simulink model "GFM1MW"  (R2024b)
settings: Solver=VariableStepAuto  StartTime=0.0  StopTime=0.5  FixedStep=0.001  MaxStep=1e-3  RelTol=1e-3
values from neighbouring files (symbols this model uses):
  Cf = 6.1509e-05    [GFM1MWParameters.m]
  fbase = 50    [GFM1MWParameters.m]
  Kffi = 0.9    [GFM1MWParameters.m]
  Kffv = 0.9    [GFM1MWParameters.m]
  Kicc = Rf/Ti    (= 50)    [GFM1MWParameters.m]
  Kiq = 0.007    [GFM1MWParameters.m]
  Kivc = k*z    [GFM1MWParameters.m]
  Kpcc = (Lf1+Lf2)/Ti    (= 3.941325)    [GFM1MWParameters.m]
  Kpvc = k    [GFM1MWParameters.m]
  Lf1 = 6.8943e-04    (= 0.00068943)    [GFM1MWParameters.m]
  Lf2 = 9.8835e-05    [GFM1MWParameters.m]
  Lth = Xth/(2*pi*fbase)    [GFM1MWParameters.m]
  Mp = (2*pi*df)/(2*Pnom)    (= 3.41477462347e-06)    [GFM1MWParameters.m]
  Nq = (Vref*dV*2)/(2*Qnom)    [GFM1MWParameters.m]
  Ppowerstep = 0e6    (= 0)    [GFM1MWParameters.m]
  Pref = 0.5e6    (= 500000)    [GFM1MWParameters.m]
  Qpowerstep = 0e6    (= 0)    [GFM1MWParameters.m]
  Qref = 0.1e6    (= 100000)    [GFM1MWParameters.m]
  Rf = 0.01    [GFM1MWParameters.m]
  Rfc = 0.3450    (= 0.345)    [GFM1MWParameters.m]
  Rth = Zth/sqrt(XtoR*XtoR+1)    [GFM1MWParameters.m]
  Rvir = 0.0293    [GFM1MWParameters.m]
  Tactivepowerstep = 1.0    (= 1)    [GFM1MWParameters.m]
  Treactivepowerstep = 1.0    (= 1)    [GFM1MWParameters.m]
  Vbase = 690    [GFM1MWParameters.m]
  Vdc = 1300    [GFM1MWParameters.m]
  Vref = Vbase*sqrt(2)/sqrt(3)    [GFM1MWParameters.m]
  w = 2*pi*fbase    (= 314.159265359)    [GFM1MWParameters.m]
  Xvir = 0.0384    [GFM1MWParameters.m]
libraries: spsSeriesRLCBranchLib x15, slpidlib x4, spsGroundLib x4, dspstat3 x4, spsabctodq0Lib x4, spsThreePhaseVIMeasurementLib x3, spsFirstOrderFilterLib x2, spsThreePhaseParallelRLCLoadLib x2, spsdq0toabcLib x1, spsDCVoltageSourceLib x1, spsPLLLib x1, spsPWMGenerator2LevelLib x1
settings Model: Creator=alexs  LastModifiedBy=sproj
settings SolverCC: ZeroCrossAlgorithm=Adaptive
settings DebuggingCC: MaskedZcDiagnostic=none  IgnoredZcDiagnostic=none

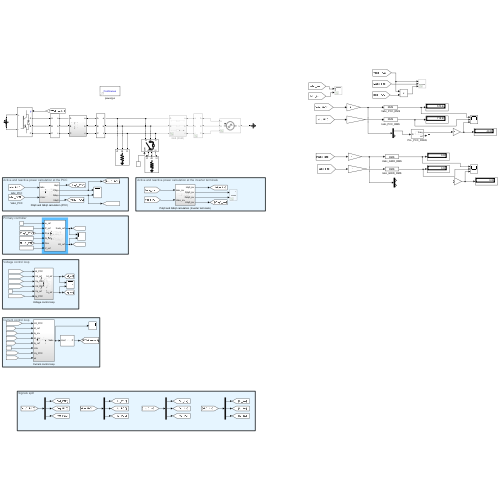
[thumbnail: Simulink's stored preview of the top-level diagram]
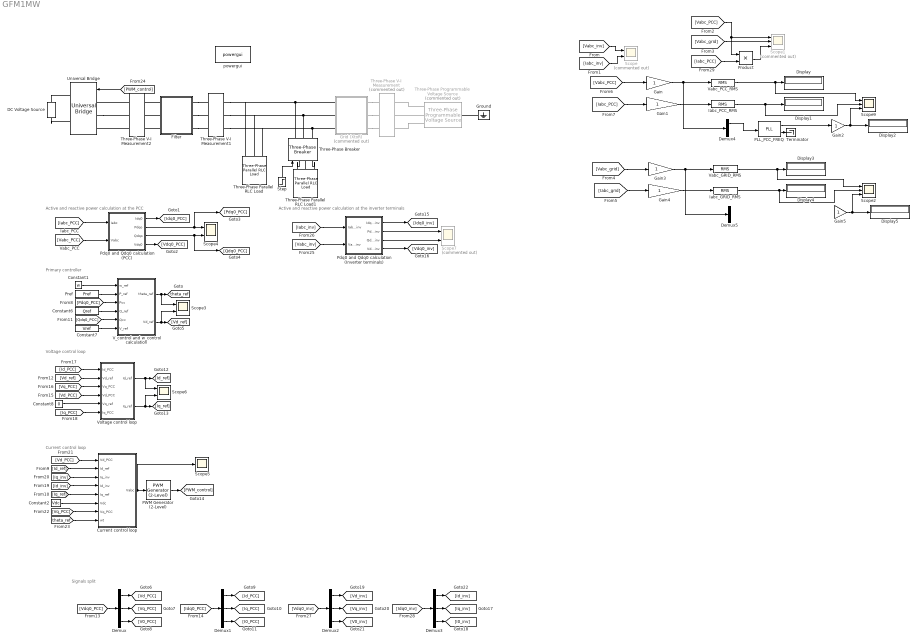
== system GFM1MW ==
  note: Active and reactive power calculation at the inverter terminals
  note: Voltage control loop
  note: Primary controller
  note: Active and reactive power calculation at the PCC
  note: Signals split
  note: Current control loop
  Constant1 : Constant  Value=w
  Constant2 : Constant  Value=Vdc
  Constant6 : Constant  Value=Qref
  Constant7 : Constant  Value=Vref
  Constant8 : Constant  Value=0
  Current control loop : Subsystem
  DC Voltage Source : spsDCVoltageSourceLib/DC Voltage Source  Amplitude=Vdc  Measurements=None
  Demux{,1..3} (4 alike) : Demux  Outputs=3
  Demux4 : Demux  Outputs=2
  Demux5 : Demux  Outputs=2
  Display{,1..5} (6 alike) : Display
      settings: Format=bank
  Filter : Subsystem
  Gain{,1..5} (6 alike) : Gain
  Grid (XtoR) : Subsystem  Commented=on
  Ground : spsGroundLib/Ground  LConnTagsString=a
  Iabc_GRID_RMS : dspstat3/RMS  run=off  directionMode=Each column  dimension=1  InputProcessing=Columns as channels (frame based)  reset_popup=None
  Iabc_PCC_RMS : dspstat3/RMS  run=off  directionMode=Each column  dimension=1  InputProcessing=Columns as channels (frame based)  reset_popup=None
  PLL_PCC_FREQ : spsPLLLib/PLL  Fmin=45  Par_Init=[0, 50]  ParK=[180, 3200, 1]  TcD=1e-4  MaxRateChangeFreq=12  FilterCutOffFreq=25  Ts=0  AGC=on
      settings: LibrarySourceBlock=sps_lib/Control/PLL
  PWM Generator (2-Level) : spsPWMGenerator2LevelLib/PWM Generator (2-Level)  ModulatorType=Three-phase bridge (6 pulses)  ModulatorMode=Unsynchronized  Fc=fsw  Pc=0  nF=27  MinMax="[ -1  1]"  SamplingTechnique=Natural  ModulatingSignals=off  m=0.8  Freq=60  Phase=0  Ts=1e-6  ShowCarrierOutport=off
  Pdq0 and Qdq0 calculation (Inverter terminals) : Subsystem
  Pdq0 and Qdq0 calculation (PCC) : Subsystem
  Pref : Constant  Value=Pref
  Product : Product
  Scope : Scope  Commented=on  NumInputPorts=2
  Scope1 : Scope  Commented=on  NumInputPorts=3
  Scope2 : Scope  NumInputPorts=3
  Scope3 : Scope  NumInputPorts=2
  Scope4 : Scope  NumInputPorts=2
  Scope5 : Scope
  Scope6 : Scope  NumInputPorts=2
  Scope7 : Scope  Commented=on  NumInputPorts=2
  Scope9 : Scope  NumInputPorts=3
  Step : Step  Time=0.1  SampleTime=0
  Terminator : Terminator
  Three-Phase Parallel RLC Load : spsThreePhaseParallelRLCLoadLib/Three-Phase Parallel RLC Load  LConnTagsString=A|B|C  Configuration=Y (grounded)  NominalVoltage=Vbase  Vabc=[1e3 1e3 1e3]  Vabcp=[1e3 1e3 1e3]  NominalFrequency=fbase  UnbalancedPower=off  ActivePower=Pref  InductivePower=Qload  CapacitivePower=0  Pabc=[10e3 9e3 11e3]  QLabc=[100 90 110]  QCabc=[100 90 110]  Pabcp=[10e3 9e3 11e3]  QLabcp=[100 90 110]  QCabcp=[100 90 110]  Measurements=None  LoadType=constant Z
  Three-Phase Parallel RLC Load1 : spsThreePhaseParallelRLCLoadLib/Three-Phase Parallel RLC Load  LConnTagsString=A|B|C  Configuration=Y (grounded)  NominalVoltage=Vbase  Vabc=[1e3 1e3 1e3]  Vabcp=[1e3 1e3 1e3]  NominalFrequency=fbase  UnbalancedPower=off  ActivePower=1e5  InductivePower=Qload  CapacitivePower=0  Pabc=[10e3 9e3 11e3]  QLabc=[100 90 110]  QCabc=[100 90 110]  Pabcp=[10e3 9e3 11e3]  QLabcp=[100 90 110]  QCabcp=[100 90 110]  Measurements=None  LoadType=constant Z
  Three-Phase Programmable Voltage Source : spsThreePhaseProgrammableVoltageSourceLib/Three-Phase Programmable Voltage Source  Commented=on  PositiveSequence="[Vbase  90 fbase]"  VariationEntity=Amplitude  VariationType=Step  VariationTypeAlt=Step  VariationStep=-0.12  VariationRate=10  VariationMagnitude=0.3  VariationFrequency=2  VariationTiming=[1 3]  VariationPhaseA=off  Amplitudes=[1 0.8 1.2 1.0]  TimeValues=[0 0.1 0.15 0.2]  HarmonicGeneration=off  HarmonicA=[3 0.2 -25 0]  HarmonicB=[2 0.15 35 2]  Timing="[0.05  3]"  BusType=swing  Pref=0  Qref=0  Qmin=-inf  Qmax=inf
  Three-Phase V-I Measurement : spsThreePhaseVIMeasurementLib/Three-Phase V-I Measurement  Commented=on  VoltageMeasurement=phase-to-ground  SetLabelV=on  LabelV=Vabc_grid  Vpu=off  VpuLL=off  CurrentMeasurement=yes  SetLabelI=on  LabelI=Iabc_grid  Ipu=off  Pbase=10000  Vbase=Vac  OutputType=Complex  PhasorSimulation=off  PSBequivalent=0
  Three-Phase V-I Measurement1 : spsThreePhaseVIMeasurementLib/Three-Phase V-I Measurement  VoltageMeasurement=phase-to-ground  SetLabelV=on  LabelV=Vabc_PCC  Vpu=off  VpuLL=off  CurrentMeasurement=yes  SetLabelI=on  LabelI=Iabc_PCC  Ipu=off  Pbase=10000  Vbase=Vac  OutputType=Complex  PhasorSimulation=off  PSBequivalent=0
  Three-Phase V-I Measurement2 : spsThreePhaseVIMeasurementLib/Three-Phase V-I Measurement  VoltageMeasurement=phase-to-ground  SetLabelV=on  LabelV=Vabc_inv  Vpu=off  VpuLL=off  CurrentMeasurement=yes  SetLabelI=on  LabelI=Iabc_inv  Ipu=off  Pbase=10000  Vbase=Vac  OutputType=Complex  PhasorSimulation=off  PSBequivalent=0
  Three-Phase Breaker : spsThreePhaseBreakerLib/Three-Phase Breaker  InitialState=open  SwitchA=on  SwitchB=on  SwitchC=on  SwitchTimes="[1/60  5/60]"  External=on  BreakerResistance=0.01  SnubberResistance=1e6  SnubberCapacitance=inf  Measurements=None
  Universal Bridge : spsUniversalBridgeLib/Universal Bridge  Arms=3  SnubberResistance=1e5  SnubberCapacitance=inf  Device=IGBT / Diodes  Ron=0  Lon=0  ForwardVoltages="[  0  0  ]"  ForwardVoltage=0  GTOparameters=[ 10e-6 , 20e-6 ]  IGBTparameters=[ 1e-6 , 2e-6 ]  Measurements=None  Measurements_2=None  converterType=Rectifier
  V_control and w_control calculation : Subsystem
  Vabc_GRID_RMS : dspstat3/RMS  run=off  directionMode=Each column  dimension=1  InputProcessing=Columns as channels (frame based)  reset_popup=None
  Vabc_PCC_RMS : dspstat3/RMS  run=off  directionMode=Each column  dimension=1  InputProcessing=Columns as channels (frame based)  reset_popup=None
  Voltage control loop : Subsystem
  powergui : sps_lib/powergui  Priority=1  SimulationMode=Continuous  SampleTime=50e-6  frequency=50  Iterations=50  frequencyindice=0  Pbase=100e6  ErrMax=1e-4  UnitsV=kV  UnitsW=MW  buscounter=0  FunctionMessages=off  echomessages=off  EnableUseOfTLC=off  CurrentSourceSwitches=off  DisableSnubberDevices=off  DisableRonSwitches=off  DisableVfSwitches=off  DisplayEquations=off  AutomaticDiscreteSolvers=off  SolverType=Tustin/Backward Euler (TBE)  Interpol=off  ExternalGateDelay=off  methode=off  Ts=10  x0status=blocks  SPID=on  SwTol=0  HookPort=off  NonlinearTolerance=1e-4  nMaxIteration=100  ContinueOnMaxIteration=off  RestoreLinks=warning  ResistiveCurrentMeasurement=off  Frange=[0:2:500]  Ylog=off  Xlog=on  ShowGrid=off  save=off  variable=ZData  structure=0  ZoomFFT=off  StartTime=0.0  cycles=1  DisplayStyle=1  fundamental=60  FreqAxis=off  MaxFrequency=1000  frequencyindicesteady=1  RmsSteady=1  display=off
  tag scope: theta_ref=global
  wires:
  [Vabc_inv] -> Scope/1
  [Iabc_inv] -> Scope/2
  [Vabc_grid] -> Scope1/2
  [Vabc_PCC] -> Product/1, Scope1/1
  Pdq0 and Qdq0 calculation (PCC)/1(Idq0) -> [Idq0_PCC]
  Pdq0 and Qdq0 calculation (PCC)/4(Vdq0) -> [Vdq0_PCC]
  Pdq0 and Qdq0 calculation (PCC)/2(Pdqo) -> Scope4/1, [Pdq0_PCC]
  Pdq0 and Qdq0 calculation (PCC)/3(Qdqo) -> [Qdq0_PCC], Scope4/2
  [Vabc_PCC] -> Gain/1
  [Iabc_PCC] -> Gain1/1
  [Iabc_PCC] -> Pdq0 and Qdq0 calculation (PCC)/1(Iabc)
  [Vabc_PCC] -> Pdq0 and Qdq0 calculation (PCC)/2(Vabc)
  Constant1/1 -> V_control and w_control calculation/1(w_ref)
  Pref/1 -> V_control and w_control calculation/2(P_ref)
  Constant6/1 -> V_control and w_control calculation/4(Q_ref)
  Constant7/1 -> V_control and w_control calculation/6(V_ref)
  V_control and w_control calculation/2(Vd_ref) -> Scope3/2, [Vd_ref]
  [Vdq0_PCC] -> Demux/1
  Demux/1 -> [Vd_PCC]
  Demux/2 -> [Vq_PCC]
  Demux/3 -> [V0_PCC]
  Demux1/1 -> [Id_PCC]
  [Idq0_PCC] -> Demux1/1
  Demux1/3 -> [I0_PCC]
  Demux1/2 -> [Iq_PCC]
  [Id_PCC] -> Voltage control loop/1(Id_PCC)
  [Vd_ref] -> Voltage control loop/2(Vd_ref)
  [Vq_PCC] -> Voltage control loop/3(Vq_PCC)
  [Vd_PCC] -> Voltage control loop/4(Vd_PCC)
  Constant8/1 -> Voltage control loop/5(Vq_ref)
  [Iq_PCC] -> Voltage control loop/6(Iq_PCC)
  Voltage control loop/1(Id_ref) -> Scope6/1, [Id_ref]
  Voltage control loop/2(Iq_ref) -> Scope6/2, [Iq_ref]
  [Vabc_inv] -> Pdq0 and Qdq0 calculation (Inverter terminals)/2(Vabc_inv)
  [Iabc_inv] -> Pdq0 and Qdq0 calculation (Inverter terminals)/1(Iabc_inv)
  Pdq0 and Qdq0 calculation (Inverter terminals)/1(Idq0_inv) -> [Idq0_inv]
  Pdq0 and Qdq0 calculation (Inverter terminals)/4(Vdq0_inv) -> [Vdq0_inv]
  Demux2/1 -> [Vd_inv]
  Demux3/2 -> [Iq_inv]
  Demux3/3 -> [I0_inv]
  [Idq0_inv] -> Demux3/1
  [Vdq0_inv] -> Demux2/1
  Demux2/3 -> [V0_inv]
  Demux3/1 -> [Id_inv]
  Demux2/2 -> [Vq_inv]
  Pdq0 and Qdq0 calculation (Inverter terminals)/2(Pdq0_inv) -> Scope7/1
  Pdq0 and Qdq0 calculation (Inverter terminals)/3(Qdq0_inv) -> Scope7/2
  [Vd_PCC] -> Current control loop/1(Vd_PCC)
  [Id_ref] -> Current control loop/2(Id_ref)
  [Iq_inv] -> Current control loop/3(Iq_inv)
  [Id_inv] -> Current control loop/4(Id_inv)
  [Iq_ref] -> Current control loop/5(Iq_ref)
  Constant2/1 -> Current control loop/6(Vdc)
  [Vq_PCC] -> Current control loop/7(Vq_PCC)
  [theta_ref] -> Current control loop/8(wt)
  Current control loop/1(Vabc) -> Scope5/1, PWM Generator (2-Level)/1
  [Qdq0_PCC] -> V_control and w_control calculation/5(Qcc)
  [Pdq0_PCC] -> V_control and w_control calculation/3(Pcc)
  V_control and w_control calculation/1(theta_ref) -> [theta_ref], Scope3/1
  PWM Generator (2-Level)/1 -> [PWM_control]
  Step/1 -> Three-Phase Breaker/1
  PLL_PCC_FREQ/2 -> Terminator/1
  Demux4/1 -> PLL_PCC_FREQ/1
  PLL_PCC_FREQ/1 -> Gain2/1
  Vabc_PCC_RMS/1 -> Scope9/1, Display/1
  Gain2/1 -> Display2/1, Scope9/3
  Product/1 -> Scope1/3
  Gain/1 -> Vabc_PCC_RMS/1, Demux4/1
  Gain1/1 -> Iabc_PCC_RMS/1
  Gain4/1 -> Iabc_GRID_RMS/1
  Gain5/1 -> Display5/1, Scope2/3
  [Iabc_grid] -> Gain4/1
  Iabc_GRID_RMS/1 -> Scope2/2, Display4/1
  [Vabc_grid] -> Gain3/1
  Vabc_GRID_RMS/1 -> Scope2/1, Display3/1
  Gain3/1 -> Vabc_GRID_RMS/1, Demux5/1
  [PWM_control] -> Universal Bridge/1
  [Iabc_PCC] -> Product/2
  Iabc_PCC_RMS/1 -> Scope9/2, Display1/1
  connections:
  Three-Phase Breaker/RConn2 -- Three-Phase V-I Measurement1/RConn2 -- Three-Phase Parallel RLC Load/LConn2 -- Grid (XtoR)/LConn2
  Three-Phase Programmable Voltage Source/RConn1 -- Three-Phase V-I Measurement/LConn1
  Three-Phase Programmable Voltage Source/RConn2 -- Three-Phase V-I Measurement/LConn2
  Three-Phase Programmable Voltage Source/RConn3 -- Three-Phase V-I Measurement/LConn3
  Three-Phase V-I Measurement2/LConn1 -- Universal Bridge/LConn1
  Three-Phase V-I Measurement2/LConn3 -- Universal Bridge/LConn3
  Universal Bridge/LConn2 -- Three-Phase V-I Measurement2/LConn2
  DC Voltage Source/RConn1 -- Universal Bridge/RConn1
  DC Voltage Source/LConn1 -- Universal Bridge/RConn2
  Three-Phase Parallel RLC Load1/LConn1 -- Three-Phase Breaker/LConn1
  Three-Phase Parallel RLC Load1/LConn2 -- Three-Phase Breaker/LConn2
  Three-Phase Parallel RLC Load1/LConn3 -- Three-Phase Breaker/LConn3
  Filter/RConn2 -- Three-Phase V-I Measurement1/LConn2
  Filter/RConn1 -- Three-Phase V-I Measurement1/LConn1
  Filter/RConn3 -- Three-Phase V-I Measurement1/LConn3
  Filter/LConn3 -- Three-Phase V-I Measurement2/RConn3
  Filter/LConn2 -- Three-Phase V-I Measurement2/RConn2
  Filter/LConn1 -- Three-Phase V-I Measurement2/RConn1
  Grid (XtoR)/RConn1 -- Three-Phase V-I Measurement/RConn1
  Grid (XtoR)/RConn2 -- Three-Phase V-I Measurement/RConn2
  Grid (XtoR)/RConn3 -- Three-Phase V-I Measurement/RConn3
  Three-Phase Breaker/RConn1 -- Three-Phase V-I Measurement1/RConn1 -- Three-Phase Parallel RLC Load/LConn1 -- Grid (XtoR)/LConn1
  Three-Phase Breaker/RConn3 -- Three-Phase Parallel RLC Load/LConn3 -- Three-Phase V-I Measurement1/RConn3 -- Grid (XtoR)/LConn3
  Ground/LConn1 -- Three-Phase Programmable Voltage Source/LConn1

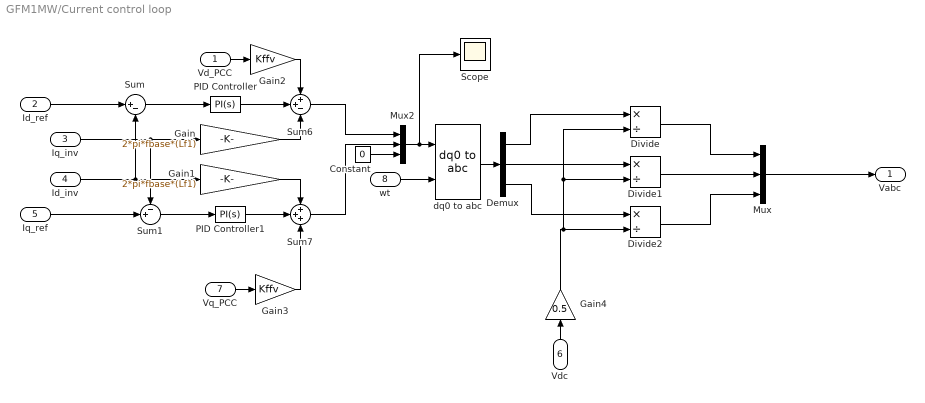
== system GFM1MW/Current control loop ==
  Vd_PCC : Inport
  Id_ref : Inport  Port=2
  Iq_inv : Inport  Port=3
  Id_inv : Inport  Port=4
  Iq_ref : Inport  Port=5
  Vdc : Inport  Port=6
  Vq_PCC : Inport  Port=7
  wt : Inport  Port=8
  Constant : Constant  Value=0
  Demux : Demux  Outputs=3
  Divide : Product  Inputs=*/
  Divide1 : Product  Inputs=*/
  Divide2 : Product  Inputs=*/
  Gain : Gain  Gain=2*pi*fbase*(Lf1)
  Gain1 : Gain  Gain=2*pi*fbase*(Lf1)
  Gain2 : Gain  Gain=Kffv
  Gain3 : Gain  Gain=Kffv
  Gain4 : Gain  Gain=0.5
  Mux : Mux  Inputs=3
  Mux2 : Mux  Inputs=3
  PID Controller : slpidlib/PID Controller  Controller=PI  Form=Parallel  TimeDomain=Continuous-time  UseExternalTs=off  SampleTime=-1  IntegratorMethod=Forward Euler  FilterMethod=Forward Euler  ControllerParametersSource=internal  P=Kpcc  I=Kicc  UseKiTs=off  D=0  UseExternalDerivativeSource=off  N=100  UseFilter=on  TunerSelectOption=Transfer Function Based (PID Tuner App)  InitialConditionSource=internal  InitialConditionForIntegrator=0  InitialConditionForFilter=0  DifferentiatorICPrevScaledInput=0  ExternalReset=none  TrackingMode=off  Kt=1  LimitOutput=off  SatLimitsSource=internal  UpperSaturationLimit=inf  LowerSaturationLimit=-inf  LinearizeAsGain=on  AntiWindupMode=none  Kb=1  LimitIntegrator=off  UpperIntegratorSaturationLimit=inf  LowerIntegratorSaturationLimit=-inf  POutMin=[]  POutMax=[]  IOutMin=[]  IOutMax=[]  DOutMin=[]  DOutMax=[]  NOutMin=[]  NOutMax=[]  SumOutMin=[]  SumOutMax=[]  SaturationOutMin=[]  SaturationOutMax=[]  PParamMin=[]  PParamMax=[]  IParamMin=[]  IParamMax=[]  DParamMin=[]  DParamMax=[]  NParamMin=[]  NParamMax=[]  KbParamMin=[]  KbParamMax=[]  KtParamMin=[]  KtParamMax=[]  KbOutMin=[]  KbOutMax=[]  KtOutMin=[]  KtOutMax=[]  IntegratorOutMin=[]  IntegratorOutMax=[]  FilterOutMin=[]  FilterOutMax=[]  SumI1OutMin=[]  SumI1OutMax=[]  SumI2OutMin=[]  SumI2OutMax=[]  SumI3OutMin=[]  SumI3OutMax=[]  SumI4OutMin=[]  SumI4OutMax=[]  SumDOutMin=[]  SumDOutMax=[]  DifferentiatorOutMin=[]  DifferentiatorOutMax=[]  FilterDiffOutCoefMin=[]  FilterDiffOutCoefMax=[]  ReciprocalOutMin=[]  ReciprocalOutMax=[]  SumDenOutMin=[]  SumDenOutMax=[]  SumNumOutMin=[]  SumNumOutMax=[]  DivideOutMin=[]  DivideOutMax=[]  UdiffTsProdOutMin=[]  UdiffTsProdOutMax=[]  NTsProdOutMin=[]  NTsProdOutMax=[]  UintegralTsProdOutMin=[]  UintegralTsProdOutMax=[]  UngainTsProdOutMin=[]  UngainTsProdOutMax=[]  ClampingZeroOutDataTypeStr=Inherit: Inherit via back propagation  ClampingZeroOutMin=[]  ClampingZeroOutMax=[]  FilterDenConstantOutDataTypeStr=Inherit: Inherit via back propagation  FilterDenConstantOutMin=[]  FilterDenConstantOutMax=[]  PCopyOutDataTypeStr=Inherit: Inherit via back propagation  PCopyOutMin=[]  PCopyOutMax=[]  NCopyOutDataTypeStr=Inherit: Inherit via back propagation  NCopyOutMin=[]  NCopyOutMax=[]  IntegratorContinuousStateAttributes=''  IntegratorStateMustResolveToSignalObject=off  IntegratorRTWStateStorageClass=Auto  FilterContinuousStateAttributes=''  FilterStateMustResolveToSignalObject=off  FilterRTWStateStorageClass=Auto  ParallelPVariant=InternalParameters  IdealPVariant=Disabled  IVariant=InternalParameters  DVariant=Disabled  IntegratorVariant=Continuous  SatVariant=Disabled  AWVariant=Passthrough  PCopyVariant=Disabled  TRVariant=Disabled  FdbkBlocksVariant=Forward  IdealPFdbkVariant=Disabled  SatFdbkVariant=Disabled  DerivativeFilterVariant=Disabled  NVariant=Disabled  NCopyVariant=Disabled_SignalSpec  FilterICVariant=Disabled  IntegratorICVariant=InternalICs  ExternalResetVariant=Disabled  TRSumVariant=Passthrough  SumFdbkVariant=Disabled  SumVariant=Sum_PI  TsampFilterVariant=InternalTs  TsampNgainVariant=Passthrough  TsampIntegralVariant=Disabled_SignalSpec  ExternalSaturationOutDataTypeStr=Inherit: Same as second input  DerivativeSourceVariant=Disabled  PreIntVariant=InternalPreInt
  PID Controller1 : slpidlib/PID Controller  Controller=PI  Form=Parallel  TimeDomain=Continuous-time  UseExternalTs=off  SampleTime=-1  IntegratorMethod=Forward Euler  FilterMethod=Forward Euler  ControllerParametersSource=internal  P=Kpcc  I=Kicc  UseKiTs=off  D=0  UseExternalDerivativeSource=off  N=100  UseFilter=on  TunerSelectOption=Transfer Function Based (PID Tuner App)  InitialConditionSource=internal  InitialConditionForIntegrator=0  InitialConditionForFilter=0  DifferentiatorICPrevScaledInput=0  ExternalReset=none  TrackingMode=off  Kt=1  LimitOutput=off  SatLimitsSource=internal  UpperSaturationLimit=inf  LowerSaturationLimit=-inf  LinearizeAsGain=on  AntiWindupMode=none  Kb=1  LimitIntegrator=off  UpperIntegratorSaturationLimit=inf  LowerIntegratorSaturationLimit=-inf  POutMin=[]  POutMax=[]  IOutMin=[]  IOutMax=[]  DOutMin=[]  DOutMax=[]  NOutMin=[]  NOutMax=[]  SumOutMin=[]  SumOutMax=[]  SaturationOutMin=[]  SaturationOutMax=[]  PParamMin=[]  PParamMax=[]  IParamMin=[]  IParamMax=[]  DParamMin=[]  DParamMax=[]  NParamMin=[]  NParamMax=[]  KbParamMin=[]  KbParamMax=[]  KtParamMin=[]  KtParamMax=[]  KbOutMin=[]  KbOutMax=[]  KtOutMin=[]  KtOutMax=[]  IntegratorOutMin=[]  IntegratorOutMax=[]  FilterOutMin=[]  FilterOutMax=[]  SumI1OutMin=[]  SumI1OutMax=[]  SumI2OutMin=[]  SumI2OutMax=[]  SumI3OutMin=[]  SumI3OutMax=[]  SumI4OutMin=[]  SumI4OutMax=[]  SumDOutMin=[]  SumDOutMax=[]  DifferentiatorOutMin=[]  DifferentiatorOutMax=[]  FilterDiffOutCoefMin=[]  FilterDiffOutCoefMax=[]  ReciprocalOutMin=[]  ReciprocalOutMax=[]  SumDenOutMin=[]  SumDenOutMax=[]  SumNumOutMin=[]  SumNumOutMax=[]  DivideOutMin=[]  DivideOutMax=[]  UdiffTsProdOutMin=[]  UdiffTsProdOutMax=[]  NTsProdOutMin=[]  NTsProdOutMax=[]  UintegralTsProdOutMin=[]  UintegralTsProdOutMax=[]  UngainTsProdOutMin=[]  UngainTsProdOutMax=[]  ClampingZeroOutDataTypeStr=Inherit: Inherit via back propagation  ClampingZeroOutMin=[]  ClampingZeroOutMax=[]  FilterDenConstantOutDataTypeStr=Inherit: Inherit via back propagation  FilterDenConstantOutMin=[]  FilterDenConstantOutMax=[]  PCopyOutDataTypeStr=Inherit: Inherit via back propagation  PCopyOutMin=[]  PCopyOutMax=[]  NCopyOutDataTypeStr=Inherit: Inherit via back propagation  NCopyOutMin=[]  NCopyOutMax=[]  IntegratorContinuousStateAttributes=''  IntegratorStateMustResolveToSignalObject=off  IntegratorRTWStateStorageClass=Auto  FilterContinuousStateAttributes=''  FilterStateMustResolveToSignalObject=off  FilterRTWStateStorageClass=Auto  ParallelPVariant=InternalParameters  IdealPVariant=Disabled  IVariant=InternalParameters  DVariant=Disabled  IntegratorVariant=Continuous  SatVariant=Disabled  AWVariant=Passthrough  PCopyVariant=Disabled  TRVariant=Disabled  FdbkBlocksVariant=Forward  IdealPFdbkVariant=Disabled  SatFdbkVariant=Disabled  DerivativeFilterVariant=Disabled  NVariant=Disabled  NCopyVariant=Disabled_SignalSpec  FilterICVariant=Disabled  IntegratorICVariant=InternalICs  ExternalResetVariant=Disabled  TRSumVariant=Passthrough  SumFdbkVariant=Disabled  SumVariant=Sum_PI  TsampFilterVariant=InternalTs  TsampNgainVariant=Passthrough  TsampIntegralVariant=Disabled_SignalSpec  ExternalSaturationOutDataTypeStr=Inherit: Same as second input  DerivativeSourceVariant=Disabled  PreIntVariant=InternalPreInt
  Scope : Scope
  Sum : Sum  Inputs=|+-
  Sum1 : Sum  Inputs=-+|
  Sum6 : Sum  Inputs=++-
  Sum7 : Sum  Inputs=+++
  dq0 to abc : spsdq0toabcLib/dq0 to abc  Alignment=Aligned with phase A axis
  Vabc : Outport
  wires:
  Gain/1 -> Sum6/3
  PID Controller1/1 -> Sum7/2
  Gain2/1 -> Sum6/1
  Iq_inv/1 -> Gain/1, Sum1/1
  Sum1/1 -> PID Controller1/1
  PID Controller/1 -> Sum6/2
  Mux2/1 -> Scope/1, dq0 to abc/1
  Id_inv/1 -> Gain1/1, Sum/2
  Vq_PCC/1 -> Gain3/1
  Sum/1 -> PID Controller/1
  Iq_ref/1 -> Sum1/2
  Gain1/1 -> Sum7/1
  Gain3/1 -> Sum7/3
  Vd_PCC/1 -> Gain2/1
  wt/1 -> dq0 to abc/2
  Id_ref/1 -> Sum/1
  Sum6/1 -> Mux2/1
  Sum7/1 -> Mux2/2
  Constant/1 -> Mux2/3
  Vdc/1 -> Gain4/1
  Mux/1 -> Vabc/1
  Gain4/1 -> Divide/2, Divide1/2, Divide2/2
  Divide2/1 -> Mux/3
  Demux/1 -> Divide/1
  Demux/2 -> Divide1/1
  Divide/1 -> Mux/1
  Demux/3 -> Divide2/1
  Divide1/1 -> Mux/2
  dq0 to abc/1 -> Demux/1

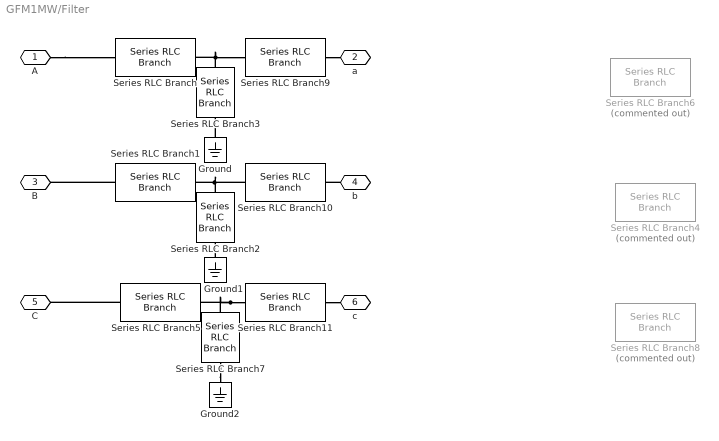
== system GFM1MW/Filter ==
  Ground : spsGroundLib/Ground  LConnTagsString=a
  Ground1 : spsGroundLib/Ground  LConnTagsString=a
  Ground2 : spsGroundLib/Ground  LConnTagsString=a
  Series RLC Branch : spsSeriesRLCBranchLib/Series RLC Branch  LConnTagsString=__new0  RConnTagsString=__new0  BranchType=RL  Resistance=Rf  Inductance=Lf1  SetiL0=off  InitialCurrent=0  Capacitance=1e-6  Setx0=off  InitialVoltage=0  Measurements=None
  Series RLC Branch1 : spsSeriesRLCBranchLib/Series RLC Branch  LConnTagsString=__new0  RConnTagsString=__new0  BranchType=RL  Resistance=Rf  Inductance=Lf1  SetiL0=off  InitialCurrent=0  Capacitance=1e-6  Setx0=off  InitialVoltage=0  Measurements=None
  Series RLC Branch10 : spsSeriesRLCBranchLib/Series RLC Branch  LConnTagsString=__new0  RConnTagsString=__new0  BranchType=L  Resistance=Rf  Inductance=Lf2  SetiL0=off  InitialCurrent=0  Capacitance=1e-6  Setx0=off  InitialVoltage=0  Measurements=None
  Series RLC Branch11 : spsSeriesRLCBranchLib/Series RLC Branch  LConnTagsString=__new0  RConnTagsString=__new0  BranchType=L  Resistance=Rf  Inductance=Lf2  SetiL0=off  InitialCurrent=0  Capacitance=1e-6  Setx0=off  InitialVoltage=0  Measurements=None
  Series RLC Branch2 : spsSeriesRLCBranchLib/Series RLC Branch  LConnTagsString=__new0  RConnTagsString=__new0  BranchType=RC  Resistance=Rfc  Inductance=1e-3  SetiL0=off  InitialCurrent=0  Capacitance=Cf  Setx0=off  InitialVoltage=0  Measurements=None
  Series RLC Branch3 : spsSeriesRLCBranchLib/Series RLC Branch  LConnTagsString=__new0  RConnTagsString=__new0  BranchType=RC  Resistance=Rfc  Inductance=1e-3  SetiL0=off  InitialCurrent=0  Capacitance=Cf  Setx0=off  InitialVoltage=0  Measurements=None
  Series RLC Branch4 : spsSeriesRLCBranchLib/Series RLC Branch  Commented=on  LConnTagsString=__new0  RConnTagsString=__new0  BranchType=L  Resistance=Rf  Inductance=Lf2  SetiL0=off  InitialCurrent=0  Capacitance=1e-6  Setx0=off  InitialVoltage=0  Measurements=None
  Series RLC Branch5 : spsSeriesRLCBranchLib/Series RLC Branch  LConnTagsString=__new0  RConnTagsString=__new0  BranchType=RL  Resistance=Rf  Inductance=Lf1  SetiL0=off  InitialCurrent=0  Capacitance=1e-6  Setx0=off  InitialVoltage=0  Measurements=None
  Series RLC Branch6 : spsSeriesRLCBranchLib/Series RLC Branch  Commented=on  LConnTagsString=__new0  RConnTagsString=__new0  BranchType=L  Resistance=Rf  Inductance=Lf2  SetiL0=off  InitialCurrent=0  Capacitance=1e-6  Setx0=off  InitialVoltage=0  Measurements=None
  Series RLC Branch7 : spsSeriesRLCBranchLib/Series RLC Branch  LConnTagsString=__new0  RConnTagsString=__new0  BranchType=RC  Resistance=Rfc  Inductance=1e-3  SetiL0=off  InitialCurrent=0  Capacitance=Cf  Setx0=off  InitialVoltage=0  Measurements=None
  Series RLC Branch8 : spsSeriesRLCBranchLib/Series RLC Branch  Commented=on  LConnTagsString=__new0  RConnTagsString=__new0  BranchType=L  Resistance=Rf  Inductance=Lf2  SetiL0=off  InitialCurrent=0  Capacitance=1e-6  Setx0=off  InitialVoltage=0  Measurements=None
  Series RLC Branch9 : spsSeriesRLCBranchLib/Series RLC Branch  LConnTagsString=__new0  RConnTagsString=__new0  BranchType=L  Resistance=Rf  Inductance=Lf2  SetiL0=off  InitialCurrent=0  Capacitance=1e-6  Setx0=off  InitialVoltage=0  Measurements=None
  A : PMIOPort  Side=Left
  a : PMIOPort  Port=2  Side=Right
  B : PMIOPort  Port=3  Side=Left
  b : PMIOPort  Port=4  Side=Right
  C : PMIOPort  Port=5  Side=Left
  c : PMIOPort  Port=6  Side=Right
  connections:
  Series RLC Branch1/LConn1 -- B/RConn1
  A/RConn1 -- Series RLC Branch/LConn1
  Ground/LConn1 -- Series RLC Branch3/RConn1
  Series RLC Branch5/LConn1 -- C/RConn1
  Series RLC Branch7/RConn1 -- Ground2/LConn1
  Ground1/LConn1 -- Series RLC Branch2/RConn1
  Series RLC Branch3/LConn1 -- Series RLC Branch9/LConn1 -- Series RLC Branch/RConn1
  b/RConn1 -- Series RLC Branch10/RConn1
  Series RLC Branch11/LConn1 -- Series RLC Branch5/RConn1 -- Series RLC Branch7/LConn1
  Series RLC Branch9/RConn1 -- a/RConn1
  Series RLC Branch10/LConn1 -- Series RLC Branch1/RConn1 -- Series RLC Branch2/LConn1
  Series RLC Branch11/RConn1 -- c/RConn1

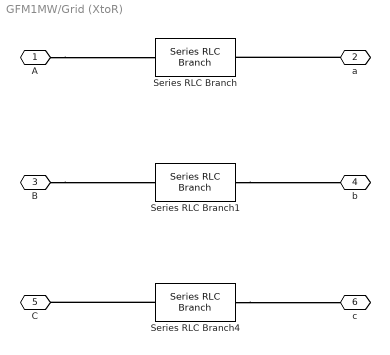
== system GFM1MW/Grid (XtoR) ==
  Series RLC Branch : spsSeriesRLCBranchLib/Series RLC Branch  LConnTagsString=__new0  RConnTagsString=__new0  BranchType=RL  Resistance=Rth  Inductance=Lth  SetiL0=off  InitialCurrent=0  Capacitance=1e-6  Setx0=off  InitialVoltage=0  Measurements=None
  Series RLC Branch1 : spsSeriesRLCBranchLib/Series RLC Branch  LConnTagsString=__new0  RConnTagsString=__new0  BranchType=RL  Resistance=Rth  Inductance=Lth  SetiL0=off  InitialCurrent=0  Capacitance=1e-6  Setx0=off  InitialVoltage=0  Measurements=None
  Series RLC Branch4 : spsSeriesRLCBranchLib/Series RLC Branch  LConnTagsString=__new0  RConnTagsString=__new0  BranchType=RL  Resistance=Rth  Inductance=Lth  SetiL0=off  InitialCurrent=0  Capacitance=1e-6  Setx0=off  InitialVoltage=0  Measurements=None
  A : PMIOPort  Side=Left
  a : PMIOPort  Port=2  Side=Right
  B : PMIOPort  Port=3  Side=Left
  b : PMIOPort  Port=4  Side=Right
  C : PMIOPort  Port=5  Side=Left
  c : PMIOPort  Port=6  Side=Right
  connections:
  B/RConn1 -- Series RLC Branch1/LConn1
  Series RLC Branch1/RConn1 -- b/RConn1
  A/RConn1 -- Series RLC Branch/LConn1
  a/RConn1 -- Series RLC Branch/RConn1
  Series RLC Branch4/RConn1 -- c/RConn1
  Series RLC Branch4/LConn1 -- C/RConn1

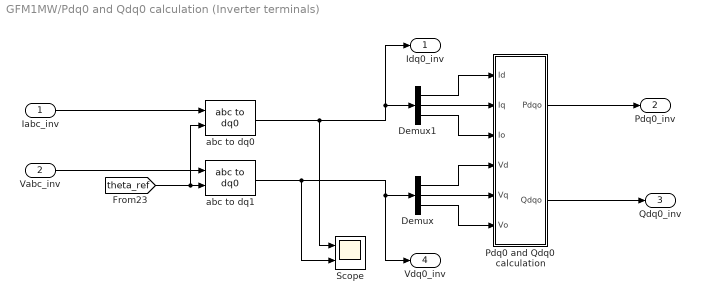
== system GFM1MW/Pdq0 and Qdq0 calculation (Inverter terminals) ==
  Iabc_inv : Inport
  Vabc_inv : Inport  Port=2
  Demux : Demux  Outputs=3
  Demux1 : Demux  Outputs=3
  Pdq0 and Qdq0 calculation : MATLAB Function  TreatAsAtomicUnit=on
  Scope : Scope  NumInputPorts=2
  abc to dq0 : spsabctodq0Lib/abc to dq0  Alignment=Aligned with phase A axis
  abc to dq1 : spsabctodq0Lib/abc to dq0  Alignment=Aligned with phase A axis
  Idq0_inv : Outport
  Pdq0_inv : Outport  Port=2
  Qdq0_inv : Outport  Port=3
  Vdq0_inv : Outport  Port=4
  wires:
  Demux1/1 -> Pdq0 and Qdq0 calculation/1(Id)
  Demux1/2 -> Pdq0 and Qdq0 calculation/2(Iq)
  Demux/2 -> Pdq0 and Qdq0 calculation/5(Vq)
  abc to dq1/1 -> Scope/2, Vdq0_inv/1, Demux/1
  Demux/1 -> Pdq0 and Qdq0 calculation/4(Vd)
  abc to dq0/1 -> Scope/1, Idq0_inv/1, Demux1/1
  Demux/3 -> Pdq0 and Qdq0 calculation/6(Vo)
  Demux1/3 -> Pdq0 and Qdq0 calculation/3(Io)
  Iabc_inv/1 -> abc to dq0/1
  Vabc_inv/1 -> abc to dq1/1
  Pdq0 and Qdq0 calculation/2(Qdqo) -> Qdq0_inv/1
  Pdq0 and Qdq0 calculation/1(Pdqo) -> Pdq0_inv/1
  [theta_ref] -> abc to dq0/2, abc to dq1/2

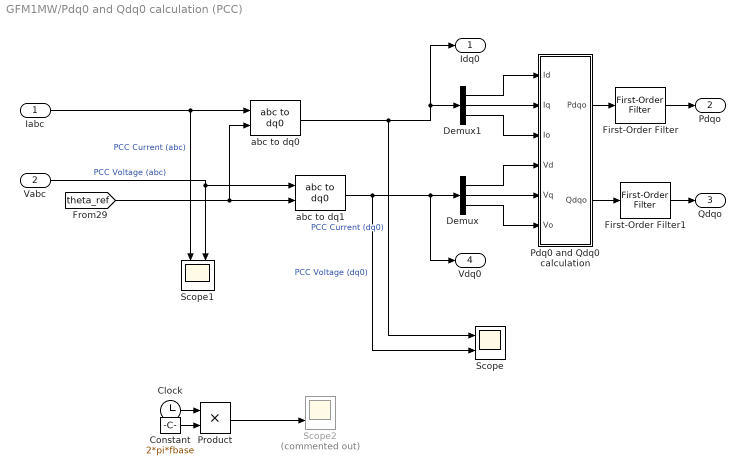
== system GFM1MW/Pdq0 and Qdq0 calculation (PCC) ==
  Iabc : Inport
  Vabc : Inport  Port=2
  Clock : Clock
  Constant : Constant  Value=2*pi*fbase
  Demux : Demux  Outputs=3
  Demux1 : Demux  Outputs=3
  First-Order Filter : spsFirstOrderFilterLib/First-Order Filter  FilterType=Lowpass  Tc=10e-3  Ts=0  Initialize=off  Vac_Init=[0, 0, 50]  Vdc_Init=0  PlotResponse=off  FreqRange="[0,  200,  1]"
  First-Order Filter1 : spsFirstOrderFilterLib/First-Order Filter  FilterType=Lowpass  Tc=10e-3  Ts=0  Initialize=off  Vac_Init=[0, 0, 50]  Vdc_Init=0  PlotResponse=off  FreqRange="[0,  200,  1]"
  Pdq0 and Qdq0 calculation : MATLAB Function  TreatAsAtomicUnit=on
  Product : Product
  Scope : Scope  NumInputPorts=2
  Scope1 : Scope  NumInputPorts=2
  Scope2 : Scope  Commented=on  NumInputPorts=2
  abc to dq0 : spsabctodq0Lib/abc to dq0  Alignment=Aligned with phase A axis
  abc to dq1 : spsabctodq0Lib/abc to dq0  Alignment=Aligned with phase A axis
  Idq0 : Outport
  Pdqo : Outport  Port=2
  Qdqo : Outport  Port=3
  Vdq0 : Outport  Port=4
  wires:
  Demux1/1 -> Pdq0 and Qdq0 calculation/1(Id)
  Demux1/2 -> Pdq0 and Qdq0 calculation/2(Iq)
  Demux/2 -> Pdq0 and Qdq0 calculation/5(Vq)
  abc to dq1/1 -> Scope/2, Vdq0/1, Demux/1  "PCC Voltage (dq0)"
  Demux/1 -> Pdq0 and Qdq0 calculation/4(Vd)
  abc to dq0/1 -> Scope/1, Idq0/1, Demux1/1  "PCC Current (dq0)"
  Demux/3 -> Pdq0 and Qdq0 calculation/6(Vo)
  Demux1/3 -> Pdq0 and Qdq0 calculation/3(Io)
  Constant/1 -> Product/2
  Clock/1 -> Product/1
  Product/1 -> Scope2/2
  [theta_ref] -> abc to dq0/2, abc to dq1/2
  Iabc/1 -> abc to dq0/1, Scope1/1  "PCC Current (abc)"
  Vabc/1 -> abc to dq1/1, Scope1/2  "PCC Voltage (abc)"
  First-Order Filter1/1 -> Qdqo/1
  Pdq0 and Qdq0 calculation/1(Pdqo) -> First-Order Filter/1
  Pdq0 and Qdq0 calculation/2(Qdqo) -> First-Order Filter1/1
  First-Order Filter/1 -> Pdqo/1

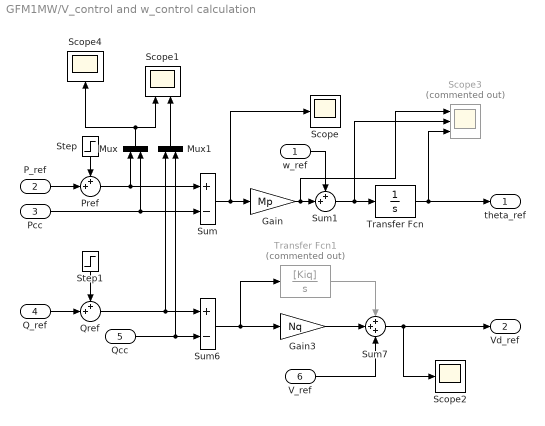
== system GFM1MW/V_control and w_control calculation ==
  w_ref : Inport
  P_ref : Inport  Port=2
  Pcc : Inport  Port=3
  Q_ref : Inport  Port=4
  Qcc : Inport  Port=5
  V_ref : Inport  Port=6
  Gain : Gain  Gain=Mp
  Gain3 : Gain  Gain=Nq
  Mux : Mux  Inputs=2
  Mux1 : Mux  Inputs=2
  Pref : Sum  Inputs=++|
  Qref : Sum  Inputs=++|
  Scope : Scope
  Scope1 : Scope  NumInputPorts=2
  Scope2 : Scope
  Scope3 : Scope  Commented=on  NumInputPorts=3
  Scope4 : Scope
  Step : Step  Time=Tactivepowerstep  After=Ppowerstep  SampleTime=0
  Step1 : Step  Time=Treactivepowerstep  After=Qpowerstep  SampleTime=0
  Sum : Sum  Inputs=+-
  Sum1 : Sum  Inputs=++|
  Sum6 : Sum  Inputs=+-
  Sum7 : Sum  Inputs=+++
  Transfer Fcn : TransferFcn  Denominator=[1 0]
  Transfer Fcn1 : TransferFcn  Commented=on  Numerator=[Kiq]  Denominator=[1 0]
  theta_ref : Outport
  Vd_ref : Outport  Port=2
  wires:
  Sum6/1 -> Transfer Fcn1/1, Gain3/1
  Sum7/1 -> Scope2/1, Vd_ref/1
  Transfer Fcn/1 -> Scope3/3, theta_ref/1
  Sum/1 -> Scope/1, Gain/1
  Sum1/1 -> Scope3/2, Transfer Fcn/1
  Gain/1 -> Scope3/1, Sum1/2
  w_ref/1 -> Sum1/1
  V_ref/1 -> Sum7/3
  Gain3/1 -> Sum7/2
  Transfer Fcn1/1 -> Sum7/1
  Qcc/1 -> Mux1/2, Sum6/2
  Pcc/1 -> Sum/2, Mux/2
  P_ref/1 -> Pref/2
  Pref/1 -> Sum/1, Mux/1
  Step/1 -> Pref/1
  Qref/1 -> Mux1/1, Sum6/1
  Q_ref/1 -> Qref/2
  Step1/1 -> Qref/1
  Mux/1 -> Scope4/1, Scope1/1
  Mux1/1 -> Scope1/2

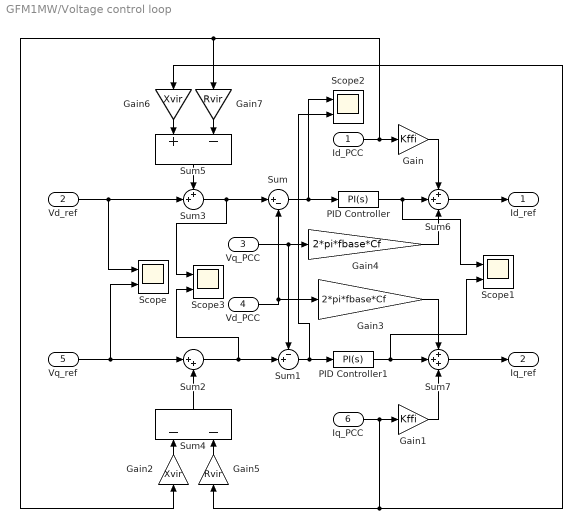
== system GFM1MW/Voltage control loop ==
  Id_PCC : Inport
  Vd_ref : Inport  Port=2
  Vq_PCC : Inport  Port=3
  Vd_PCC : Inport  Port=4
  Vq_ref : Inport  Port=5
  Iq_PCC : Inport  Port=6
  Gain : Gain  Gain=Kffi
  Gain1 : Gain  Gain=Kffi
  Gain2 : Gain  Gain=Xvir
  Gain3 : Gain  Gain=2*pi*fbase*Cf
  Gain4 : Gain  Gain=2*pi*fbase*Cf
  Gain5 : Gain  Gain=Rvir
  Gain6 : Gain  Gain=Xvir
  Gain7 : Gain  Gain=Rvir
  PID Controller : slpidlib/PID Controller  Controller=PI  Form=Parallel  TimeDomain=Continuous-time  UseExternalTs=off  SampleTime=-1  IntegratorMethod=Forward Euler  FilterMethod=Forward Euler  ControllerParametersSource=internal  P=Kpvc  I=Kivc  UseKiTs=off  D=0  UseExternalDerivativeSource=off  N=100  UseFilter=on  TunerSelectOption=Transfer Function Based (PID Tuner App)  InitialConditionSource=internal  InitialConditionForIntegrator=0  InitialConditionForFilter=0  DifferentiatorICPrevScaledInput=0  ExternalReset=none  TrackingMode=off  Kt=1  LimitOutput=off  SatLimitsSource=internal  UpperSaturationLimit=inf  LowerSaturationLimit=-inf  LinearizeAsGain=on  AntiWindupMode=none  Kb=1  LimitIntegrator=off  UpperIntegratorSaturationLimit=inf  LowerIntegratorSaturationLimit=-inf  POutMin=[]  POutMax=[]  IOutMin=[]  IOutMax=[]  DOutMin=[]  DOutMax=[]  NOutMin=[]  NOutMax=[]  SumOutMin=[]  SumOutMax=[]  SaturationOutMin=[]  SaturationOutMax=[]  PParamMin=[]  PParamMax=[]  IParamMin=[]  IParamMax=[]  DParamMin=[]  DParamMax=[]  NParamMin=[]  NParamMax=[]  KbParamMin=[]  KbParamMax=[]  KtParamMin=[]  KtParamMax=[]  KbOutMin=[]  KbOutMax=[]  KtOutMin=[]  KtOutMax=[]  IntegratorOutMin=[]  IntegratorOutMax=[]  FilterOutMin=[]  FilterOutMax=[]  SumI1OutMin=[]  SumI1OutMax=[]  SumI2OutMin=[]  SumI2OutMax=[]  SumI3OutMin=[]  SumI3OutMax=[]  SumI4OutMin=[]  SumI4OutMax=[]  SumDOutMin=[]  SumDOutMax=[]  DifferentiatorOutMin=[]  DifferentiatorOutMax=[]  FilterDiffOutCoefMin=[]  FilterDiffOutCoefMax=[]  ReciprocalOutMin=[]  ReciprocalOutMax=[]  SumDenOutMin=[]  SumDenOutMax=[]  SumNumOutMin=[]  SumNumOutMax=[]  DivideOutMin=[]  DivideOutMax=[]  UdiffTsProdOutMin=[]  UdiffTsProdOutMax=[]  NTsProdOutMin=[]  NTsProdOutMax=[]  UintegralTsProdOutMin=[]  UintegralTsProdOutMax=[]  UngainTsProdOutMin=[]  UngainTsProdOutMax=[]  ClampingZeroOutDataTypeStr=Inherit: Inherit via back propagation  ClampingZeroOutMin=[]  ClampingZeroOutMax=[]  FilterDenConstantOutDataTypeStr=Inherit: Inherit via back propagation  FilterDenConstantOutMin=[]  FilterDenConstantOutMax=[]  PCopyOutDataTypeStr=Inherit: Inherit via back propagation  PCopyOutMin=[]  PCopyOutMax=[]  NCopyOutDataTypeStr=Inherit: Inherit via back propagation  NCopyOutMin=[]  NCopyOutMax=[]  IntegratorContinuousStateAttributes=''  IntegratorStateMustResolveToSignalObject=off  IntegratorRTWStateStorageClass=Auto  FilterContinuousStateAttributes=''  FilterStateMustResolveToSignalObject=off  FilterRTWStateStorageClass=Auto  ParallelPVariant=InternalParameters  IdealPVariant=Disabled  IVariant=InternalParameters  DVariant=Disabled  IntegratorVariant=Continuous  SatVariant=Disabled  AWVariant=Passthrough  PCopyVariant=Disabled  TRVariant=Disabled  FdbkBlocksVariant=Forward  IdealPFdbkVariant=Disabled  SatFdbkVariant=Disabled  DerivativeFilterVariant=Disabled  NVariant=Disabled  NCopyVariant=Disabled_SignalSpec  FilterICVariant=Disabled  IntegratorICVariant=InternalICs  ExternalResetVariant=Disabled  TRSumVariant=Passthrough  SumFdbkVariant=Disabled  SumVariant=Sum_PI  TsampFilterVariant=InternalTs  TsampNgainVariant=Passthrough  TsampIntegralVariant=Disabled_SignalSpec  ExternalSaturationOutDataTypeStr=Inherit: Same as second input  DerivativeSourceVariant=Disabled  PreIntVariant=InternalPreInt
  PID Controller1 : slpidlib/PID Controller  Controller=PI  Form=Parallel  TimeDomain=Continuous-time  UseExternalTs=off  SampleTime=-1  IntegratorMethod=Forward Euler  FilterMethod=Forward Euler  ControllerParametersSource=internal  P=Kpvc  I=Kivc  UseKiTs=off  D=0  UseExternalDerivativeSource=off  N=100  UseFilter=on  TunerSelectOption=Transfer Function Based (PID Tuner App)  InitialConditionSource=internal  InitialConditionForIntegrator=0  InitialConditionForFilter=0  DifferentiatorICPrevScaledInput=0  ExternalReset=none  TrackingMode=off  Kt=1  LimitOutput=off  SatLimitsSource=internal  UpperSaturationLimit=inf  LowerSaturationLimit=-inf  LinearizeAsGain=on  AntiWindupMode=none  Kb=1  LimitIntegrator=off  UpperIntegratorSaturationLimit=inf  LowerIntegratorSaturationLimit=-inf  POutMin=[]  POutMax=[]  IOutMin=[]  IOutMax=[]  DOutMin=[]  DOutMax=[]  NOutMin=[]  NOutMax=[]  SumOutMin=[]  SumOutMax=[]  SaturationOutMin=[]  SaturationOutMax=[]  PParamMin=[]  PParamMax=[]  IParamMin=[]  IParamMax=[]  DParamMin=[]  DParamMax=[]  NParamMin=[]  NParamMax=[]  KbParamMin=[]  KbParamMax=[]  KtParamMin=[]  KtParamMax=[]  KbOutMin=[]  KbOutMax=[]  KtOutMin=[]  KtOutMax=[]  IntegratorOutMin=[]  IntegratorOutMax=[]  FilterOutMin=[]  FilterOutMax=[]  SumI1OutMin=[]  SumI1OutMax=[]  SumI2OutMin=[]  SumI2OutMax=[]  SumI3OutMin=[]  SumI3OutMax=[]  SumI4OutMin=[]  SumI4OutMax=[]  SumDOutMin=[]  SumDOutMax=[]  DifferentiatorOutMin=[]  DifferentiatorOutMax=[]  FilterDiffOutCoefMin=[]  FilterDiffOutCoefMax=[]  ReciprocalOutMin=[]  ReciprocalOutMax=[]  SumDenOutMin=[]  SumDenOutMax=[]  SumNumOutMin=[]  SumNumOutMax=[]  DivideOutMin=[]  DivideOutMax=[]  UdiffTsProdOutMin=[]  UdiffTsProdOutMax=[]  NTsProdOutMin=[]  NTsProdOutMax=[]  UintegralTsProdOutMin=[]  UintegralTsProdOutMax=[]  UngainTsProdOutMin=[]  UngainTsProdOutMax=[]  ClampingZeroOutDataTypeStr=Inherit: Inherit via back propagation  ClampingZeroOutMin=[]  ClampingZeroOutMax=[]  FilterDenConstantOutDataTypeStr=Inherit: Inherit via back propagation  FilterDenConstantOutMin=[]  FilterDenConstantOutMax=[]  PCopyOutDataTypeStr=Inherit: Inherit via back propagation  PCopyOutMin=[]  PCopyOutMax=[]  NCopyOutDataTypeStr=Inherit: Inherit via back propagation  NCopyOutMin=[]  NCopyOutMax=[]  IntegratorContinuousStateAttributes=''  IntegratorStateMustResolveToSignalObject=off  IntegratorRTWStateStorageClass=Auto  FilterContinuousStateAttributes=''  FilterStateMustResolveToSignalObject=off  FilterRTWStateStorageClass=Auto  ParallelPVariant=InternalParameters  IdealPVariant=Disabled  IVariant=InternalParameters  DVariant=Disabled  IntegratorVariant=Continuous  SatVariant=Disabled  AWVariant=Passthrough  PCopyVariant=Disabled  TRVariant=Disabled  FdbkBlocksVariant=Forward  IdealPFdbkVariant=Disabled  SatFdbkVariant=Disabled  DerivativeFilterVariant=Disabled  NVariant=Disabled  NCopyVariant=Disabled_SignalSpec  FilterICVariant=Disabled  IntegratorICVariant=InternalICs  ExternalResetVariant=Disabled  TRSumVariant=Passthrough  SumFdbkVariant=Disabled  SumVariant=Sum_PI  TsampFilterVariant=InternalTs  TsampNgainVariant=Passthrough  TsampIntegralVariant=Disabled_SignalSpec  ExternalSaturationOutDataTypeStr=Inherit: Same as second input  DerivativeSourceVariant=Disabled  PreIntVariant=InternalPreInt
  Scope{,1..3} (4 alike) : Scope  NumInputPorts=2
  Sum : Sum  Inputs=|+-
  Sum1 : Sum  Inputs=-+|
  Sum2 : Sum  Inputs=|++
  Sum3 : Sum  Inputs=++|
  Sum4 : Sum  Inputs=--
  Sum5 : Sum  Inputs=+-
  Sum6 : Sum  Inputs=++-
  Sum7 : Sum  Inputs=+++
  Id_ref : Outport
  Iq_ref : Outport  Port=2
  wires:
  Vq_PCC/1 -> Gain4/1, Sum1/1
  PID Controller1/1 -> Scope1/2, Sum7/2
  Gain3/1 -> Sum7/1
  Sum1/1 -> Scope2/2, PID Controller1/1
  Vd_PCC/1 -> Sum/2, Gain3/1
  Gain4/1 -> Sum6/3
  PID Controller/1 -> Scope1/1, Sum6/2
  Sum7/1 -> Iq_ref/1
  Sum6/1 -> Id_ref/1
  Gain/1 -> Sum6/1
  Gain1/1 -> Sum7/3
  Vq_ref/1 -> Sum2/1, Scope/2
  Sum2/1 -> Scope3/2, Sum1/2
  Vd_ref/1 -> Sum3/2, Scope/1
  Sum3/1 -> Scope3/1, Sum/1
  Gain2/1 -> Sum4/1
  Gain5/1 -> Sum4/2
  Id_PCC/1 -> Gain2/1, Gain7/1, Gain/1
  Iq_PCC/1 -> Gain5/1, Gain6/1, Gain1/1
  Gain6/1 -> Sum5/1
  Gain7/1 -> Sum5/2
  Sum/1 -> Scope2/1, PID Controller/1
  Sum5/1 -> Sum3/1
  Sum4/1 -> Sum2/2

== matlab function GFM1MW/Pdq0 and Qdq0 calculation (PCC)/Pdq0 and Qdq0 calculation ==
  data: Pdqo output; Id input; Iq input; Io input; Vd input; Vq input; Vo input; Qdqo output
function [Pdqo,Qdqo]= fcn(Id,Iq,Io,Vd,Vq,Vo)

% Power in dq0 system
Pdqo=(3/2)*(Vd*Id+Vq*Iq+2*Vo);
Qdqo=(3/2)*(Vq*Id-Vd*Iq);

== matlab function GFM1MW/Pdq0 and Qdq0 calculation (Inverter terminals)/Pdq0 and Qdq0 calculation ==
  data: Pdqo output; Id input; Iq input; Io input; Vd input; Vq input; Vo input; Qdqo output
function [Pdqo,Qdqo]= fcn(Id,Iq,Io,Vd,Vq,Vo)

% Power in dq0 system
Pdqo=(3/2)*(Vd*Id+Vq*Iq+2*Vo);
Qdqo=(3/2)*(Vq*Id-Vd*Iq);
